simulink model "Stockton_Project1_model"  (R2014a)
settings: Solver=ode23  StartTime=0.0  StopTime=20  FixedStep=0.2  RelTol=1e-10
values from neighbouring files (symbols this model uses):
  den = conv(CE_lp,CE_sp)    [Final.m]    (also in Fuzzy_PID_Comp.m = dens{i}; Stockton_Project1.m = [230.6,2508,2161,1406,63.04,32.01])
  num = -4.516*conv([1 -0.008],[1 0.506])    [Final.m]    (also in Fuzzy_PID_Comp.m = nums{i}; Stockton_Project1.m = [3361,1357,102.2])
  scalar = 25    [Fuzzy_PID_Comp.m]
undefined symbols (not defined in the file or in its folder): data0, data1, data2
settings Model: Creator=nick  LastModifiedBy=nick
settings SolverCC: ZeroCrossControl=DisableAll  ZeroCrossAlgorithm=Adaptive
settings DebuggingCC: SolverPrmCheckMsg=none

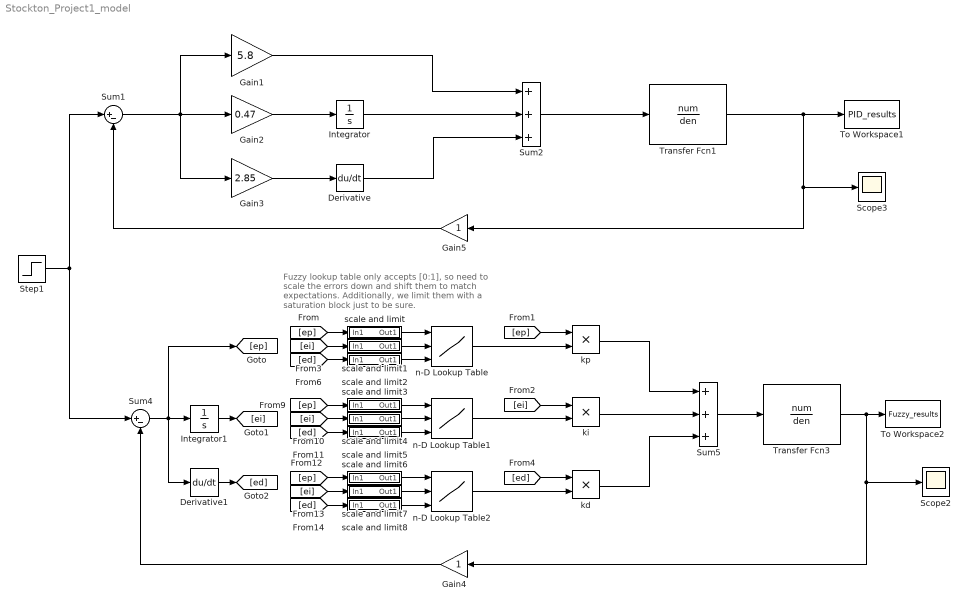
== system Stockton_Project1_model ==
  note: Fuzzy lookup table only accepts [0:1], so
      | need to scale the errors down and shift them to
      | match expectations. Additionally, we limit them
      | with a saturation block just to be sure.
  Derivative : Derivative
  Derivative1 : Derivative
  Gain1 : Gain  Gain=5.8
  Gain2 : Gain  Gain=0.47
  Gain3 : Gain  Gain=2.85
  Gain4 : Gain
  Gain5 : Gain
  Integrator : Integrator
  Integrator1 : Integrator
  Scope2 : Scope
      settings: YMin=-0.1  YMax=1.1  SaveName=ScopeData2
  Scope3 : Scope
      settings: SaveName=ScopeData3
  Step1 : Step  Time=0  SampleTime=0
  Sum1 : Sum  Inputs=|+-
  Sum2 : Sum  Inputs=+++
  Sum4 : Sum  Inputs=|+-
  Sum5 : Sum  Inputs=+++
  To Workspace1 : ToWorkspace  VariableName=PID_results  SaveFormat=Timeseries  SampleTime=-1
  To Workspace2 : ToWorkspace  VariableName=Fuzzy_results  SaveFormat=Timeseries  SampleTime=-1
  Transfer Fcn1 : TransferFcn  Numerator=num  Denominator=den
  Transfer Fcn3 : TransferFcn  Numerator=num  Denominator=den
  kd : Product
  ki : Product
  kp : Product
  n-D Lookup Table : Lookup_n-D  NumberOfTableDimensions=3  BreakpointsForDimension1=0:0.01:1  BreakpointsForDimension2=0:0.01:1  BreakpointsForDimension3=0:0.01:1  Table=data0  InternalRulePriority=Speed  RndMeth=Simplest  InputSameDT=on
  n-D Lookup Table1 : Lookup_n-D  NumberOfTableDimensions=3  BreakpointsForDimension1=0:0.01:1  BreakpointsForDimension2=0:0.01:1  BreakpointsForDimension3=0:0.01:1  Table=data1  InternalRulePriority=Speed  RndMeth=Simplest  InputSameDT=on
  n-D Lookup Table2 : Lookup_n-D  NumberOfTableDimensions=3  BreakpointsForDimension1=0:0.01:1  BreakpointsForDimension2=0:0.01:1  BreakpointsForDimension3=0:0.01:1  Table=data2  InternalRulePriority=Speed  RndMeth=Simplest  InputSameDT=on
  scale and limit : Subsystem
  scale and limit1 : Subsystem
  scale and limit2 : Subsystem
  scale and limit3 : Subsystem
  scale and limit4 : Subsystem
  scale and limit5 : Subsystem
  scale and limit6 : Subsystem
  scale and limit7 : Subsystem
  scale and limit8 : Subsystem
  wires:
  Step1/1 -> Sum1/1, Sum4/1
  Transfer Fcn1/1 -> To Workspace1/1, Gain5/1, Scope3/1
  Gain1/1 -> Sum2/1
  Sum1/1 -> Gain3/1, Gain2/1, Gain1/1
  Gain4/1 -> Sum4/2
  [ep] -> scale and limit/1(In1)
  [ei] -> scale and limit1/1(In1)
  [ed] -> scale and limit2/1(In1)
  [ep] -> scale and limit3/1(In1)
  [ei] -> scale and limit4/1(In1)
  [ed] -> scale and limit5/1(In1)
  [ep] -> scale and limit6/1(In1)
  [ei] -> scale and limit7/1(In1)
  [ed] -> scale and limit8/1(In1)
  n-D Lookup Table/1 -> kp/2
  [ep] -> kp/1
  n-D Lookup Table1/1 -> ki/2
  [ei] -> ki/1
  n-D Lookup Table2/1 -> kd/2
  [ed] -> kd/1
  kd/1 -> Sum5/3
  ki/1 -> Sum5/2
  kp/1 -> Sum5/1
  Sum4/1 -> [ep], Derivative1/1, Integrator1/1
  Integrator1/1 -> [ei]
  Derivative1/1 -> [ed]
  scale and limit/1(Out1) -> n-D Lookup Table/1
  scale and limit8/1(Out1) -> n-D Lookup Table2/3
  scale and limit7/1(Out1) -> n-D Lookup Table2/2
  scale and limit6/1(Out1) -> n-D Lookup Table2/1
  scale and limit5/1(Out1) -> n-D Lookup Table1/3
  scale and limit4/1(Out1) -> n-D Lookup Table1/2
  scale and limit3/1(Out1) -> n-D Lookup Table1/1
  scale and limit2/1(Out1) -> n-D Lookup Table/3
  scale and limit1/1(Out1) -> n-D Lookup Table/2
  Sum5/1 -> Transfer Fcn3/1
  Transfer Fcn3/1 -> Gain4/1, Scope2/1, To Workspace2/1
  Sum2/1 -> Transfer Fcn1/1
  Gain3/1 -> Derivative/1
  Derivative/1 -> Sum2/3
  Gain2/1 -> Integrator/1
  Integrator/1 -> Sum2/2
  Gain5/1 -> Sum1/2

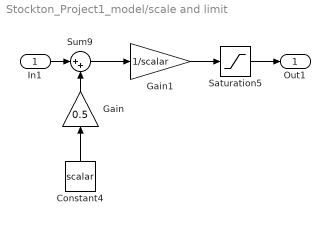
== system Stockton_Project1_model/scale and limit ==
  In1 : Inport
  Constant4 : Constant  Value=scalar
  Gain : Gain  Gain=0.5
  Gain1 : Gain  Gain=1/scalar
  Saturation5 : Saturate  UpperLimit=1  LowerLimit=0
  Sum9 : Sum  Inputs=|++
  Out1 : Outport
  wires:
  In1/1 -> Sum9/1
  Gain1/1 -> Saturation5/1
  Sum9/1 -> Gain1/1
  Saturation5/1 -> Out1/1
  Constant4/1 -> Gain/1
  Gain/1 -> Sum9/2

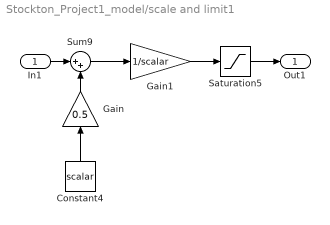
== system Stockton_Project1_model/scale and limit1 ==
  In1 : Inport
  Constant4 : Constant  Value=scalar
  Gain : Gain  Gain=0.5
  Gain1 : Gain  Gain=1/scalar
  Saturation5 : Saturate  UpperLimit=1  LowerLimit=0
  Sum9 : Sum  Inputs=|++
  Out1 : Outport
  wires:
  In1/1 -> Sum9/1
  Gain1/1 -> Saturation5/1
  Sum9/1 -> Gain1/1
  Saturation5/1 -> Out1/1
  Constant4/1 -> Gain/1
  Gain/1 -> Sum9/2

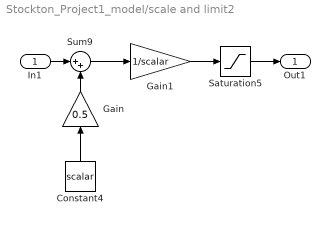
== system Stockton_Project1_model/scale and limit2 ==
  In1 : Inport
  Constant4 : Constant  Value=scalar
  Gain : Gain  Gain=0.5
  Gain1 : Gain  Gain=1/scalar
  Saturation5 : Saturate  UpperLimit=1  LowerLimit=0
  Sum9 : Sum  Inputs=|++
  Out1 : Outport
  wires:
  In1/1 -> Sum9/1
  Gain1/1 -> Saturation5/1
  Sum9/1 -> Gain1/1
  Saturation5/1 -> Out1/1
  Constant4/1 -> Gain/1
  Gain/1 -> Sum9/2

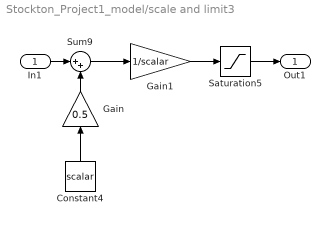
== system Stockton_Project1_model/scale and limit3 ==
  In1 : Inport
  Constant4 : Constant  Value=scalar
  Gain : Gain  Gain=0.5
  Gain1 : Gain  Gain=1/scalar
  Saturation5 : Saturate  UpperLimit=1  LowerLimit=0
  Sum9 : Sum  Inputs=|++
  Out1 : Outport
  wires:
  In1/1 -> Sum9/1
  Gain1/1 -> Saturation5/1
  Sum9/1 -> Gain1/1
  Saturation5/1 -> Out1/1
  Constant4/1 -> Gain/1
  Gain/1 -> Sum9/2

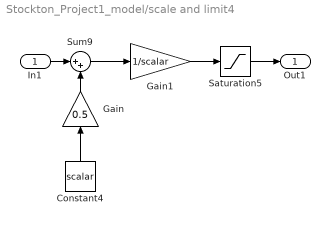
== system Stockton_Project1_model/scale and limit4 ==
  In1 : Inport
  Constant4 : Constant  Value=scalar
  Gain : Gain  Gain=0.5
  Gain1 : Gain  Gain=1/scalar
  Saturation5 : Saturate  UpperLimit=1  LowerLimit=0
  Sum9 : Sum  Inputs=|++
  Out1 : Outport
  wires:
  In1/1 -> Sum9/1
  Gain1/1 -> Saturation5/1
  Sum9/1 -> Gain1/1
  Saturation5/1 -> Out1/1
  Constant4/1 -> Gain/1
  Gain/1 -> Sum9/2

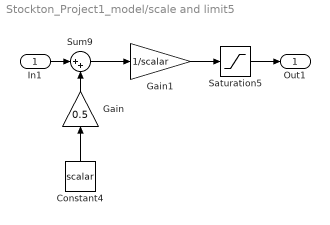
== system Stockton_Project1_model/scale and limit5 ==
  In1 : Inport
  Constant4 : Constant  Value=scalar
  Gain : Gain  Gain=0.5
  Gain1 : Gain  Gain=1/scalar
  Saturation5 : Saturate  UpperLimit=1  LowerLimit=0
  Sum9 : Sum  Inputs=|++
  Out1 : Outport
  wires:
  In1/1 -> Sum9/1
  Gain1/1 -> Saturation5/1
  Sum9/1 -> Gain1/1
  Saturation5/1 -> Out1/1
  Constant4/1 -> Gain/1
  Gain/1 -> Sum9/2

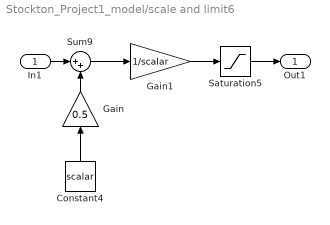
== system Stockton_Project1_model/scale and limit6 ==
  In1 : Inport
  Constant4 : Constant  Value=scalar
  Gain : Gain  Gain=0.5
  Gain1 : Gain  Gain=1/scalar
  Saturation5 : Saturate  UpperLimit=1  LowerLimit=0
  Sum9 : Sum  Inputs=|++
  Out1 : Outport
  wires:
  In1/1 -> Sum9/1
  Gain1/1 -> Saturation5/1
  Sum9/1 -> Gain1/1
  Saturation5/1 -> Out1/1
  Constant4/1 -> Gain/1
  Gain/1 -> Sum9/2

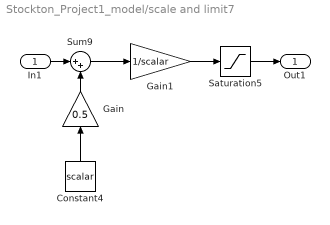
== system Stockton_Project1_model/scale and limit7 ==
  In1 : Inport
  Constant4 : Constant  Value=scalar
  Gain : Gain  Gain=0.5
  Gain1 : Gain  Gain=1/scalar
  Saturation5 : Saturate  UpperLimit=1  LowerLimit=0
  Sum9 : Sum  Inputs=|++
  Out1 : Outport
  wires:
  In1/1 -> Sum9/1
  Gain1/1 -> Saturation5/1
  Sum9/1 -> Gain1/1
  Saturation5/1 -> Out1/1
  Constant4/1 -> Gain/1
  Gain/1 -> Sum9/2

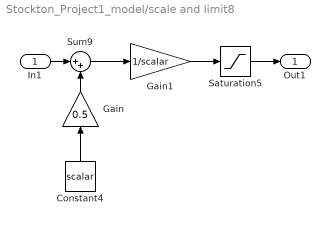
== system Stockton_Project1_model/scale and limit8 ==
  In1 : Inport
  Constant4 : Constant  Value=scalar
  Gain : Gain  Gain=0.5
  Gain1 : Gain  Gain=1/scalar
  Saturation5 : Saturate  UpperLimit=1  LowerLimit=0
  Sum9 : Sum  Inputs=|++
  Out1 : Outport
  wires:
  In1/1 -> Sum9/1
  Gain1/1 -> Saturation5/1
  Sum9/1 -> Gain1/1
  Saturation5/1 -> Out1/1
  Constant4/1 -> Gain/1
  Gain/1 -> Sum9/2
